simulink model "simulatorPNS_AGC_3"  (Simulink 7.8)
settings: Solver=ode45  StartTime=0  StopTime=Tsim  RelTol=1e-3
undefined symbols (not defined in the file): Ac, Bc, Cc, Dc, Lc
settings Model: Creator=stefano  LastModifiedBy=stefano
settings DebuggingCC: SolverPrmCheckMsg=none

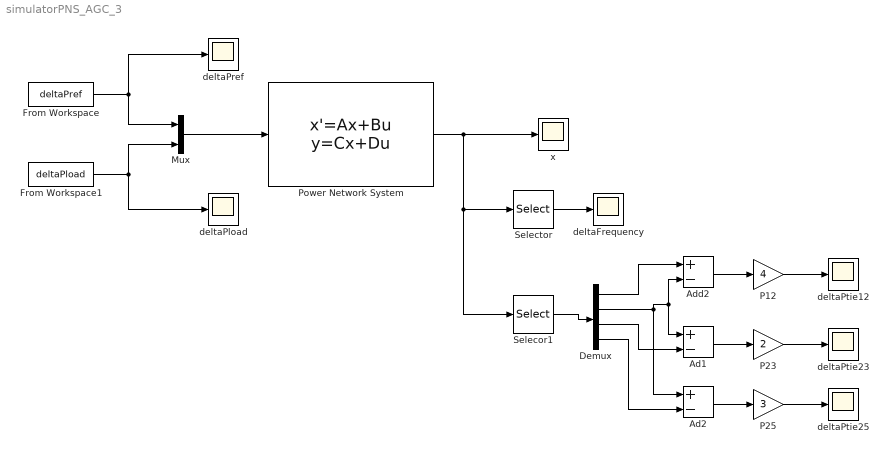
== system simulatorPNS_AGC_3 ==
  Ad1 : Sum  Inputs=+-
  Ad2 : Sum  Inputs=+-
  Add2 : Sum  Inputs=+-
  Demux : Demux
  From Workspace : FromWorkspace  VariableName=deltaPref  SampleTime=1  Interpolate=off  OutputAfterFinalValue=Holding final value
  From Workspace1 : FromWorkspace  VariableName=deltaPload  SampleTime=1  Interpolate=off  OutputAfterFinalValue=Holding final value
  Mux : Mux  Inputs=2
  P12 : Gain  Gain=4
  P23 : Gain  Gain=2
  P25 : Gain  Gain=3
  Power Network System : StateSpace  A=Ac  B=[ Bc Lc ]  C=Cc  D=[ Dc zeros(size(Cc,1),size(Lc,2)) ]
  Selecor1 : Selector  InputPortWidth=16  IndexOptions=Index vector (dialog)  Indices=1:4:size(Ac,1)  OutputSizes=1
  Selector : Selector  InputPortWidth=16  IndexOptions=Index vector (dialog)  Indices=2:4:size(Ac,1)  OutputSizes=1
  deltaFrequency : Scope
      settings: TimeRange=4.192872117400418  YMin=-0.04124040920716115  YMax=0.1762787723785165  SaveName=xxx1
  deltaPload : Scope
      settings: TimeRange=4.192872117400418  YMin=-0.04124040920716115  YMax=0.1762787723785165
  deltaPref : Scope
      settings: TimeRange=4.192872117400418  YMin=-0.04124040920716115  YMax=0.1762787723785165
  deltaPtie12 : Scope
      settings: TimeRange=4.192872117400418  YMin=-0.04124040920716115  YMax=0.1762787723785165  SaveName=xxx2
  deltaPtie23 : Scope
      settings: TimeRange=4.192872117400418  YMin=-0.04124040920716115  YMax=0.1762787723785165  SaveName=xxx3
  deltaPtie25 : Scope
      settings: TimeRange=4.192872117400418  YMin=-0.04124040920716115  YMax=0.1762787723785165  SaveName=xxx5
  x : Scope
      settings: TimeRange=4.192872117400418  YMin=-0.04124040920716115  YMax=0.1762787723785165  SaveName=xxx
  wires:
  Mux/1 -> Power Network System/1
  From Workspace1/1 -> Mux/2, deltaPload/1
  From Workspace/1 -> Mux/1, deltaPref/1
  Power Network System/1 -> x/1, Selector/1, Selecor1/1
  Selector/1 -> deltaFrequency/1
  Selecor1/1 -> Demux/1
  Add2/1 -> P12/1
  P12/1 -> deltaPtie12/1
  Ad1/1 -> P23/1
  P23/1 -> deltaPtie23/1
  Demux/1 -> Add2/1
  Demux/2 -> Add2/2, Ad1/1, Ad2/1
  Demux/3 -> Ad1/2
  Ad2/1 -> P25/1
  P25/1 -> deltaPtie25/1
  Demux/4 -> Ad2/2
